simulink model "untitled"  (R2019b)
settings: Solver=VariableStepAuto  StartTime=0.0  StopTime=10.0  RelTol=1e-3
settings Model: Creator=Tesla  LastModifiedBy=Tesla

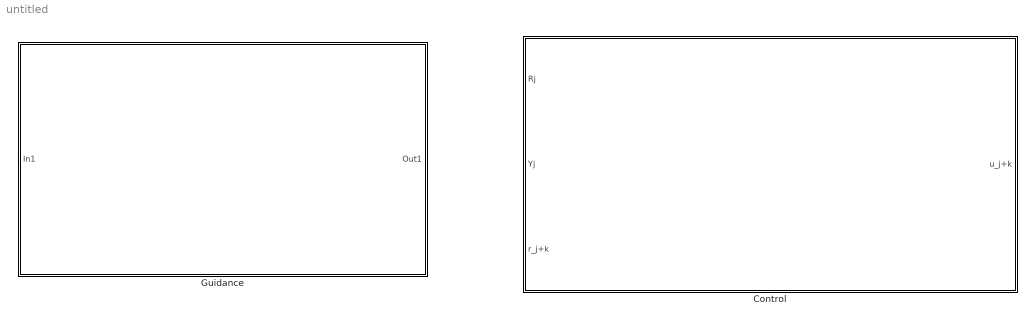
== system untitled ==
  Control : Subsystem
  Guidance : Subsystem

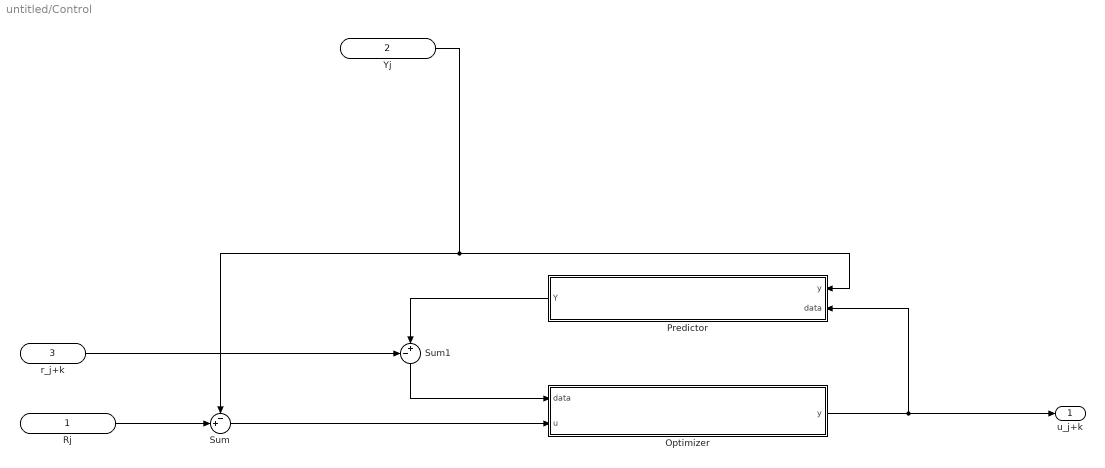
== system untitled/Control ==
  Rj : Inport
  Yj : Inport  Port=2
  r_j+k : Inport  Port=3
  Optimizer : MATLAB Function  TreatAsAtomicUnit=on
  Predictor : MATLAB Function  TreatAsAtomicUnit=on
  Sum : Sum  Inputs=-+|
  Sum1 : Sum  Inputs=-+|
  u_j+k : Outport
  wires:
  Rj/1 -> Sum/2
  Yj/1 -> Sum/1, Predictor/1(y)
  Sum/1 -> Optimizer/2(u)
  Sum1/1 -> Optimizer/1(data)
  Optimizer/1(y) -> Predictor/2(data), u_j+k/1
  Predictor/1(Y) -> Sum1/2
  r_j+k/1 -> Sum1/1

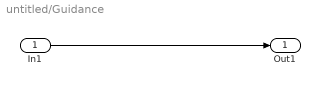
== system untitled/Guidance ==
  In1 : Inport
  Out1 : Outport
  wires:
  In1/1 -> Out1/1

== matlab function untitled/Control/Optimizer ==
  data: data input; u input; y output
function y = fcn(data, u)

y = u;

== matlab function untitled/Control/Predictor ==
  data: y input; Y output; data input
function Y = fcn(y, data)

y = u;
